simulink model "Matlab_and_Simulink"  (R2024b)
settings: Solver=FixedStepDiscrete  StartTime=0.0  StopTime=450*60  FixedStep=1  RelTol=1e-3
libraries: simulink x2
settings Model: Creator=raulp  LastModifiedBy=raulp

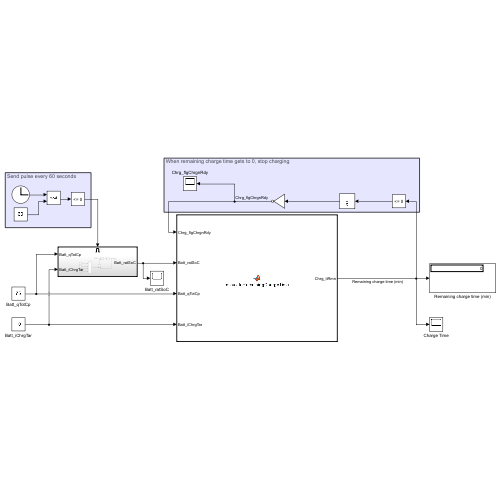
[thumbnail: Simulink's stored preview of the top-level diagram]
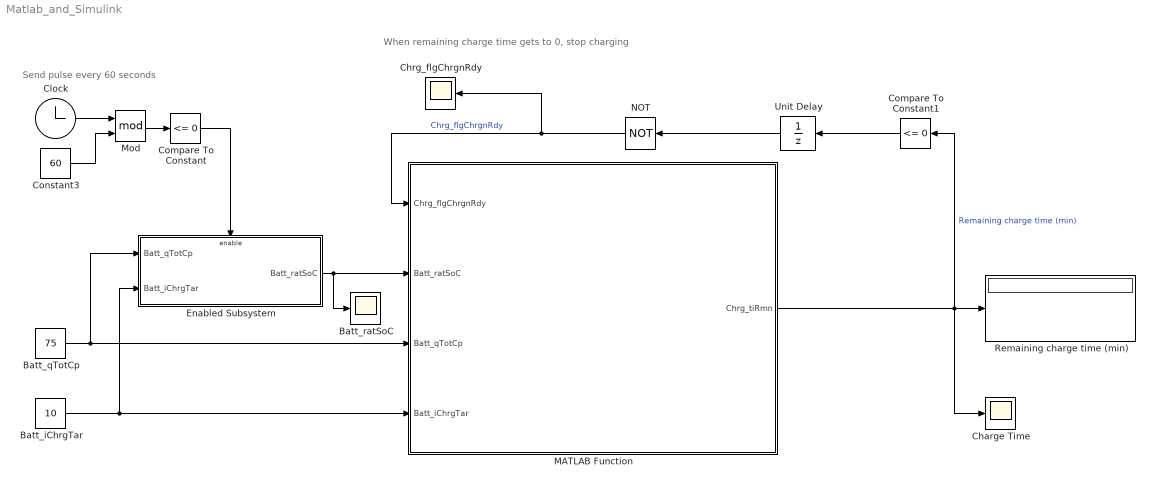
== system Matlab_and_Simulink ==
  note: When remaining charge time gets to 0, stop charging
  note: Send pulse every 60 seconds
  Batt_iChrgTar : Constant  Value=10
  Batt_qTotCp : Constant  Value=75
  Batt_ratSoC : Scope
  Charge Time : Scope
  Chrg_flgChrgnRdy : Scope
  Clock : Clock
  Compare To Constant : simulink/Logic and Bit Operations/Compare To Constant  relop=<=  const=0  OutDataTypeStr=boolean
  Compare To Constant1 : simulink/Logic and Bit Operations/Compare To Constant  relop=<=  const=0  OutDataTypeStr=boolean
  Constant3 : Constant  Value=60
  Enabled Subsystem : Subsystem  TreatAsAtomicUnit=on
  MATLAB Function : MATLAB Function  TreatAsAtomicUnit=on
  Mod : Math  Operator=mod
  NOT : Logic  Operator=NOT  IconShape=distinctive  AllPortsSameDT=off  OutDataTypeStr=boolean
  Remaining charge time (min) : Display
      settings: Format=decimal (Stored Integer)
  Unit Delay : UnitDelay  SampleTime=-1  HasFrameUpgradeWarning=on
  wires:
  MATLAB Function/1(Chrg_tiRmn) -> Charge Time/1, Remaining charge time (min)/1, Compare To Constant1/1  "Remaining charge time (min)"
  Batt_qTotCp/1 -> Enabled Subsystem/1(Batt_qTotCp), MATLAB Function/3(Batt_qTotCp)
  Batt_iChrgTar/1 -> Enabled Subsystem/2(Batt_iChrgTar), MATLAB Function/4(Batt_iChrgTar)
  Enabled Subsystem/1(Batt_ratSoC) -> Batt_ratSoC/1, MATLAB Function/2(Batt_ratSoC)
  Clock/1 -> Mod/1
  Constant3/1 -> Mod/2
  Mod/1 -> Compare To Constant/1
  Compare To Constant/1 -> Enabled Subsystem/Enable
  Compare To Constant1/1 -> Unit Delay/1
  NOT/1 -> Chrg_flgChrgnRdy/1, MATLAB Function/1(Chrg_flgChrgnRdy)  "Chrg_flgChrgnRdy"
  Unit Delay/1 -> NOT/1

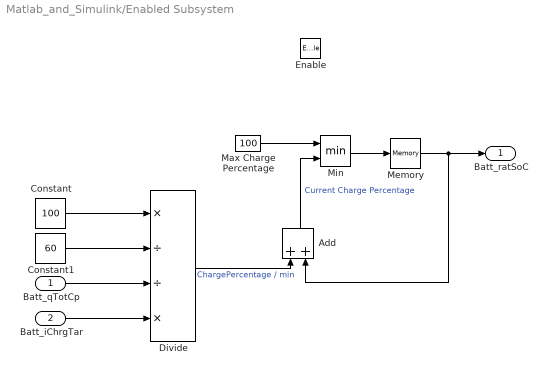
== system Matlab_and_Simulink/Enabled Subsystem ==
  Batt_qTotCp : Inport
  Batt_iChrgTar : Inport  Port=2
  Enable : EnablePort
  Add : Sum
  Constant : Constant  Value=100
  Constant1 : Constant  Value=60
  Divide : Product  Inputs=*//*
  Max Charge Percentage : Constant  Value=100
  Memory : Memory
  Min : MinMax  Inputs=2
  Batt_ratSoC : Outport
  wires:
  Memory/1 -> Batt_ratSoC/1, Add/2
  Constant/1 -> Divide/1
  Constant1/1 -> Divide/2
  Batt_qTotCp/1 -> Divide/3
  Batt_iChrgTar/1 -> Divide/4
  Divide/1 -> Add/1  "ChargePercentage / min"
  Add/1 -> Min/2  "Current Charge Percentage"
  Min/1 -> Memory/1
  Max Charge Percentage/1 -> Min/1

== matlab function Matlab_and_Simulink/MATLAB Function ==
  data: Chrg_flgChrgnRdy input; Chrg_tiRmn output; Batt_ratSoC input; Batt_qTotCp input; Batt_iChrgTar input
function Chrg_tiRmn = calculateRemainingChargeTime(Chrg_flgChrgnRdy, Batt_ratSoC, Batt_qTotCp, Batt_iChrgTar)

% Inputs:
%   Chrg_flgChrgnRdy: Charging readiness flag [boolean]
%   Batt_ratSoC: Battery state of charge [%]
%   Batt_qTotCp: Battery total capacity [Ah]
%   Batt_iChrgTar: Agreed charging current [A]

% Output:
%   Chrg_tiRmn: Remaining time for full charging [min]

    if ~Chrg_flgChrgnRdy  % Stop charging if charging flag is set to 0
        Chrg_tiRmn = 0;
        return;
    end

    remainingCapacity = (100 - Batt_ratSoC) / 100 * Batt_qTotCp;

    chargingTimeHours = remainingCapacity / Batt_iChrgTar;
    Chrg_tiRmn = chargingTimeHours * 60;

end
